simulink subsystem "MCU"  (R2023a)
settings: Solver=VariableStepAuto  StartTime=0.0  StopTime=10.0  RelTol=1e-3
model mask{PID_P=1, PID_I=1, PID_D=1, Km=1, Ke=2}
  mask prompts: Km "Motor momentum coeff"; Ke "Error gain coeff"
settings Model: Creator=user  LastModifiedBy=user

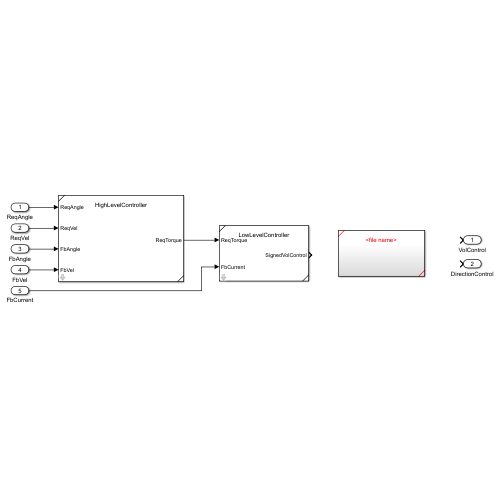
[thumbnail: Simulink's stored preview of the top-level diagram]
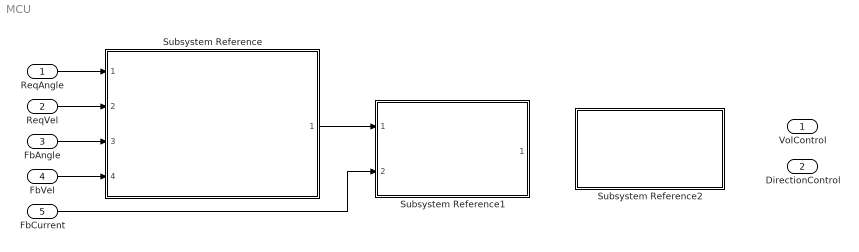
== system MCU ==
  ReqAngle : Inport
  ReqVel : Inport  Port=2
  FbAngle : Inport  Port=3
  FbVel : Inport  Port=4
  FbCurrent : Inport  Port=5
  Subsystem Reference : Subsystem  ReferencedSubsystem=HighLevelController  PID_P=PID_P  PID_I=PID_I  PID_D=PID_D
  Subsystem Reference1 : Subsystem  ReferencedSubsystem=LowLevelController  Km=Km  KLowMK=Ke
  Subsystem Reference2 : Subsystem  ReferencedSubsystem=<file name>
  VolControl : Outport
  DirectionControl : Outport  Port=2
  wires:
  ReqAngle/1 -> Subsystem Reference/1
  ReqVel/1 -> Subsystem Reference/2
  FbAngle/1 -> Subsystem Reference/3
  FbVel/1 -> Subsystem Reference/4
  Subsystem Reference/1 -> Subsystem Reference1/1
  FbCurrent/1 -> Subsystem Reference1/2

== system MCU/Subsystem Reference2 ==
